simulink library "Lib_Cntrl_LimitCntrlPI_TMATS_org"  (Simulink 10.0)
settings: Solver=ode45  StartTime=0.0  StopTime=10.0  RelTol=1e-3  EnableMultiTasking=on
undefined symbols (not defined in the file): DiscIntNeverNeededParam
Description:
  | Thomas Modules
settings Model: Creator=jwchapm2  LastModifiedBy=bhisma

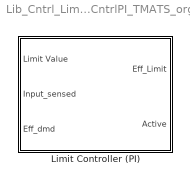
== system Lib_Cntrl_LimitCntrlPI_TMATS_org ==
  Limit Controller (PI) : Subsystem  mask(T-MATS: Limit Controller (PI)){Kp_M=1, Ki_M=1, PI_IC_M=70, WGain_M=400, Ts_M=0.1}
      mask prompts: Kp_M "Kp_M - Proportional gain"; Ki_M "Ki_M - Integral gain"; PI_IC_M "PI_IC_M - PI initial condition"; WGain_M "WGain_M - Windup protection gain"; Ts_M "Ts_M - Sample time (sec)"
      mask help: This block contains a PI controller with anti-windup protection. Gains, Kp and Ki, are defined as gains in the block.
      mask Help: web(which('Control_TMATS_LimCPI.html'),'-helpbrowser')

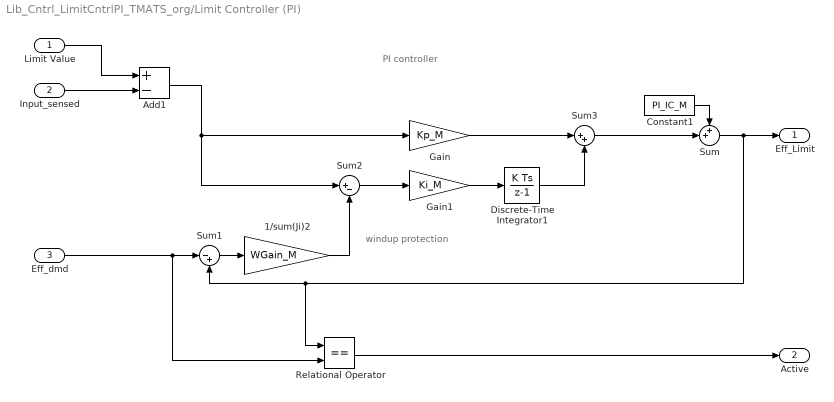
== system Lib_Cntrl_LimitCntrlPI_TMATS_org/Limit Controller (PI) ==
  note: windup protection
  note: PI controller
  Limit Value : Inport
  Input_sensed : Inport  Port=2
  Eff_dmd : Inport  Port=3
  1/sum(Ji)2 : Gain  Gain=WGain_M  SaturateOnIntegerOverflow=on  OutDataTypeStr=Inherit: Same as input  ParamDataTypeStr=Inherit: Same as input
  Add1 : Sum  Inputs=+-
  Constant1 : Constant  Value=PI_IC_M
  Discrete-Time Integrator1 : DiscreteIntegrator  SampleTime=Ts_M  ICPrevOutput=DiscIntNeverNeededParam  ICPrevScaledInput=DiscIntNeverNeededParam
  Gain : Gain  Gain=Kp_M
  Gain1 : Gain  Gain=Ki_M
  Relational Operator : RelationalOperator  Operator===  OutDataTypeStr=boolean  RndMeth=Nearest
  Sum : Sum  Inputs=++|
  Sum1 : Sum  Inputs=|-+
  Sum2 : Sum  Inputs=|+-
  Sum3 : Sum  Inputs=|++
  Eff_Limit : Outport
  Active : Outport  Port=2
  wires:
  Add1/1 -> Sum2/1, Gain/1
  Input_sensed/1 -> Add1/2
  Gain/1 -> Sum3/1
  Limit Value/1 -> Add1/1
  Discrete-Time Integrator1/1 -> Sum3/2
  Sum3/1 -> Sum/2
  Constant1/1 -> Sum/1
  Sum/1 -> Relational Operator/1, Sum1/2, Eff_Limit/1
  Eff_dmd/1 -> Relational Operator/2, Sum1/1
  Sum1/1 -> 1/sum(Ji)2/1
  1/sum(Ji)2/1 -> Sum2/2
  Sum2/1 -> Gain1/1
  Gain1/1 -> Discrete-Time Integrator1/1
  Relational Operator/1 -> Active/1
